simulink model "SimScript"  (R2018b)
settings: Solver=FixedStepAuto  StartTime=0.0  StopTime=1000  FixedStep=0.001  RelTol=1e-3
values from neighbouring files (symbols this model uses):
  cpp = 1000    [script1.m]
  CVp = cpp * rop * Vp    (= 19200)    [script1.m]
  CVw = cpp * rop * Vw    (= 24000)    [script1.m]
  dfp = 0    [script1.m]
  dt = 200    [script1.m]
  dTg = 0    [script1.m]
  dTkz = 0    [script1.m]
  dTzew = 0    [script1.m]
  fp0 = fp    (= 1.11111111111)    [script1.m]
  k1 = (Cp * TkzN - Cp * TwewN) / ((TwewN - TzewN) + 1/4 * (TpN - TgN))    (= 444.444444444)    [script1.m]
  k2 = 1/4 * k1    (= 111.111111111)    [script1.m]
  kp = 1/4 * k1 * (TpN - TgN) / (TwewN - TpN)    (= 222.222222222)    [script1.m]
  rop = 1.2    [script1.m]
  Tg0 = TgN    (= -10)    [script1.m]
  Tkz0 = TkzN    (= 35)    [script1.m]
  Tp0 = (kp * Twew0 + k2 * Tg0) / (k2 + kp)    (= 10)    [script1.m]
  Twew0 = (Cp0 * Tkz0 + k1 * Tzew0 + k2 * kp * Tg0 / (k2 + kp)) / (Cp0 + k1 + kp - kp * kp / (k2 + kp))    (= 20)    [script1.m]
  Tzew0 = TzewN    (= -20)    [script1.m]
settings Model: Creator=wojciechkonury  LastModifiedBy=wojciechkonury

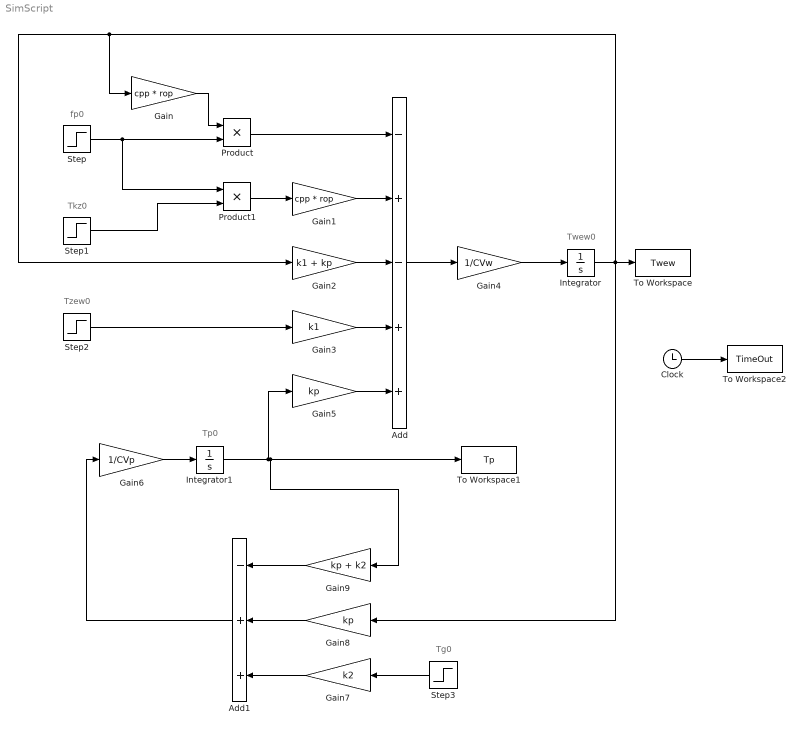
== system SimScript ==
  note: Tp0
  note: Twew0
  note: Tg0
  note: Tzew0
  note: Tkz0
  note: fp0
  Add : Sum  Inputs=-+-++
  Add1 : Sum  Inputs=-++
  Clock : Clock
  Gain : Gain  Gain=cpp * rop
  Gain1 : Gain  Gain=cpp * rop
  Gain2 : Gain  Gain=k1 + kp
  Gain3 : Gain  Gain=k1
  Gain4 : Gain  Gain=1/CVw
  Gain5 : Gain  Gain=kp
  Gain6 : Gain  Gain=1/CVp
  Gain7 : Gain  Gain=k2
  Gain8 : Gain  Gain=kp
  Gain9 : Gain  Gain=kp + k2
  Integrator : Integrator  InitialCondition=Twew0
  Integrator1 : Integrator  InitialCondition=Tp0
  Product : Product
  Product1 : Product
  Step : Step  Time=dt  Before=fp0  After=fp0 + dfp  SampleTime=0
  Step1 : Step  Time=dt  Before=Tkz0  After=Tkz0 + dTkz  SampleTime=0
  Step2 : Step  Time=dt  Before=Tzew0  After=Tzew0 + dTzew  SampleTime=0
  Step3 : Step  Time=dt  Before=Tg0  After=Tg0 + dTg  SampleTime=0
  To Workspace : ToWorkspace  VariableName=Twew  SampleTime=-1
  To Workspace1 : ToWorkspace  VariableName=Tp  SampleTime=-1
  To Workspace2 : ToWorkspace  VariableName=TimeOut  SampleTime=-1
  wires:
  Step/1 -> Product1/1, Product/2
  Gain/1 -> Product/1
  Product/1 -> Add/1
  Step1/1 -> Product1/2
  Product1/1 -> Gain1/1
  Gain1/1 -> Add/2
  Gain2/1 -> Add/3
  Step2/1 -> Gain3/1
  Gain3/1 -> Add/4
  Add/1 -> Gain4/1
  Gain4/1 -> Integrator/1
  Gain5/1 -> Add/5
  Integrator1/1 -> Gain5/1, Gain9/1, To Workspace1/1
  Gain6/1 -> Integrator1/1
  Add1/1 -> Gain6/1
  Gain7/1 -> Add1/3
  Step3/1 -> Gain7/1
  Gain8/1 -> Add1/2
  Integrator/1 -> Gain8/1, Gain2/1, Gain/1, To Workspace/1
  Gain9/1 -> Add1/1
  Clock/1 -> To Workspace2/1
